simulink subsystem "control_pulses_generator"  (R2022a)
settings: Solver=VariableStepAuto  StartTime=0.0  StopTime=0.02  RelTol=1e-3
undefined symbols (not defined in the file): PAUSE_PRD, REPEATS_PRD
settings Model: DefaultTestHarness=control_pulses_generator_harness  Creator=andre  LastModifiedBy=andre

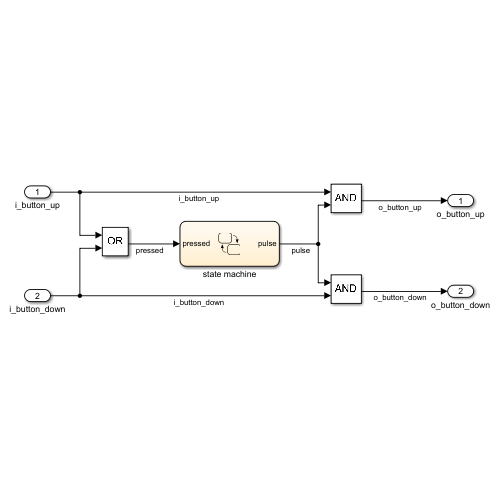
[thumbnail: Simulink's stored preview of the top-level diagram]
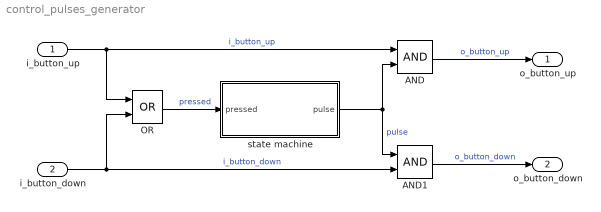
== system control_pulses_generator ==
  i_button_up : Inport  OutDataTypeStr=boolean  PortDimensions=1
  i_button_down : Inport  Port=2  OutDataTypeStr=boolean  PortDimensions=1
  AND : Logic  AllPortsSameDT=off  OutDataTypeStr=boolean
  AND1 : Logic  AllPortsSameDT=off  OutDataTypeStr=boolean
  OR : Logic  Operator=OR  AllPortsSameDT=off  OutDataTypeStr=boolean
  state machine : Stateflow chart  TreatAsAtomicUnit=on
  o_button_up : Outport  OutDataTypeStr=boolean  PortDimensions=1
  o_button_down : Outport  Port=2  OutDataTypeStr=boolean  PortDimensions=1
  wires:
  state machine/1(pulse) -> AND1/1, AND/2  "pulse"
  AND/1 -> o_button_up/1  "o_button_up"
  AND1/1 -> o_button_down/1  "o_button_down"
  OR/1 -> state machine/1(pressed)  "pressed"
  i_button_up/1 -> AND/1, OR/1  "i_button_up"
  i_button_down/1 -> OR/2, AND1/2  "i_button_down"

== stateflow chart control_pulses_generator/state machine ==
  state IDLE
    en, du:
    pulse = false;
  state PAUSE
    du:
    pulse = false;
  state REPEATS
    du:
    pulse = false;
  REPEATS -> REPEATS [order 1] : after(REPEATS_PRD, sec)
      | {pulse = true;}
  (default) -> IDLE
  PAUSE -> IDLE [order 1] : [~pressed]
  PAUSE -> REPEATS [order 2] : after(PAUSE_PRD, sec)
      | {pulse = true;}
  IDLE -> PAUSE : [pressed]
      | {pulse = true;}
  (junction 12) -> IDLE
  REPEATS -> (junction 11) [order 2] : [~pressed]
  (junction 11) -> (junction 12)
  data: pressed input boolean; pulse output boolean; REPEATS_PRD parameter; PAUSE_PRD parameter
